simulink model "localPlanServer"  (R2024a)
settings: Solver=FixedStepDiscrete  StartTime=0.0  StopTime=inf  RelTol=1e-3
model workspace (MAT data in the model file):
  SL_ROS_VariableLengthArrays_MaxSizes.CommonInfo.ArrayTruncateAction = 'EmitWarning'
  SL_ROS_VariableLengthArrays_MaxSizes.MsgTypeMap = containers.Map
  SL_ROS_VariableLengthArrays_MaxSizes.MsgTypeMap.serialization.keys = {'std_msgs/Float64MultiArray', 'std_msgs/Int8MultiArray'}
  SL_ROS_VariableLengthArrays_MaxSizes.MsgTypeMap.serialization.values{1}.PropertyName = 'data'
  SL_ROS_VariableLengthArrays_MaxSizes.MsgTypeMap.serialization.values{1}.DataType = 'double'
  SL_ROS_VariableLengthArrays_MaxSizes.MsgTypeMap.serialization.values{1}.MaxLength = 30000
  SL_ROS_VariableLengthArrays_MaxSizes.MsgTypeMap.serialization.values{2}.PropertyName = 'data'
  SL_ROS_VariableLengthArrays_MaxSizes.MsgTypeMap.serialization.values{2}.DataType = 'int8'
  SL_ROS_VariableLengthArrays_MaxSizes.MsgTypeMap.serialization.values{2}.MaxLength = 1500000
  SL_ROS_VariableLengthArrays_MaxSizes.MsgTypeMap.serialization.uniformity = 0
  SL_ROS_VariableLengthArrays_MaxSizes.MsgTypeMap.serialization.keyType = 'char'
  SL_ROS_VariableLengthArrays_MaxSizes.MsgTypeMap.serialization.valueType = 'any'
undefined symbols (not defined in the file): nearestidx, needglobalreplan, needlocalreplan, optimizedpath, timestamps, velcmds
libraries: roshelperlib x6, simulink x2, ros2lib x2
settings Model: Creator=cstabile  LastModifiedBy=cstabile
settings OptimizationCC: EnhancedBackFolding=on  PassReuseOutputArgsAs=Individual arguments  ZeroExternalMemoryAtStartup=off  ZeroInternalMemoryAtStartup=off  MaxStackSize=64  OptimizeBlockOrder=speed  DifferentSizesBufferReuse=on  OptimizationCustomize=off  EfficientTunableParamExpr=on
settings DebuggingCC: ParameterTunabilityLossMsg=error
settings SFSimCC: MATLABDynamicMemAlloc=off
settings RTWCC: Description=Embedded Coder  SystemTargetFile=ert.tlc  HardwareBoard=Robot Operating System 2 (ROS 2)  TLCOptions="-aInlineSetEventsForThisBaseRateFcn=TLC_FALSE -aSuppressMultiTaskScheduler=TLC_FALSE  -aRateBasedStepFcn=0"  TemplateMakefile=ert_default_tmf  Toolchain=Colcon Tools  TargetLang=C++
settings CodeAppCC: ForceParamTrailComments=on  IgnoreCustomStorageClasses=off  OperatorAnnotations=on  SimulinkDataObjDesc=on  SFDataObjDesc=on  InsertBlockDesc=on
settings ERTTargetCC: CodeInterfacePackaging=C++ class  RootIOFormat=Structure reference

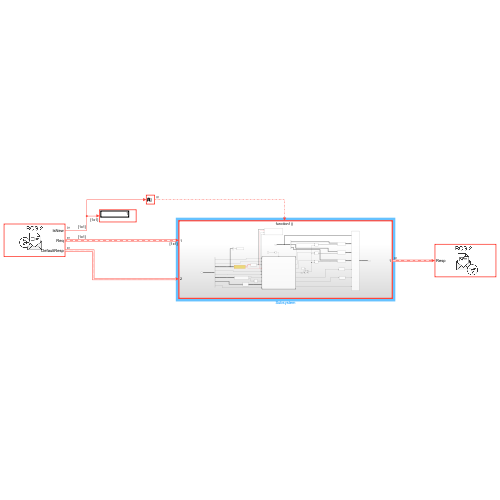
[thumbnail: Simulink's stored preview of the top-level diagram]
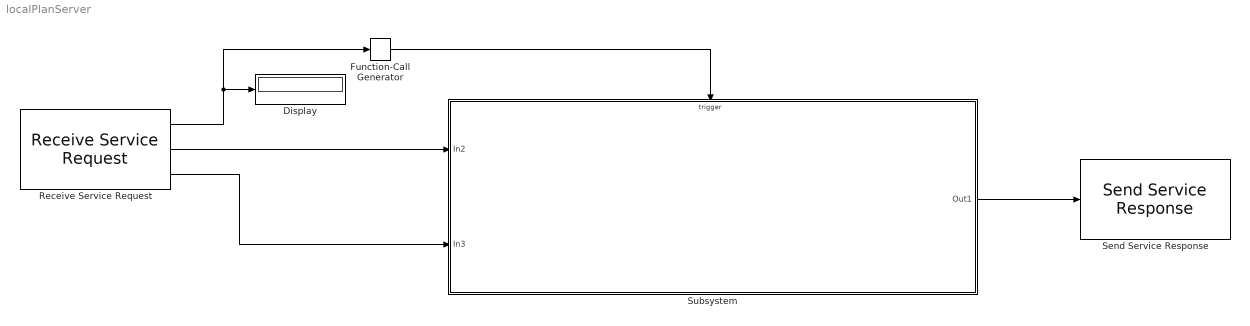
== system localPlanServer ==
  Display : Display
  Function-Call Generator : simulink/Ports & Subsystems/Function-Call Generator  sample_time=1  numberOfIterations=1  DisallowWideOutput=off  ShowEnablePort=on
  Receive Service Request : ros2lib/Receive Service Request  service=/planLocal  serviceType=offroad_msg/PlanLocal  SampleTime=-1  ShowDefaultRespOutput=on  BlockId=ServRec_localPlanServer_1  QOSHistory=Keep last  QOSDepth=1  QOSReliability=Reliable  QOSDurability=Volatile  QOSDeadline=Inf  QOSLifespan=Inf  QOSLiveliness=Automatic  QOSLeaseDuration=Inf  QOSAvoidROSNamespaceConventions=off
      settings: LibrarySourceBlock=ros2lib/Receive Request
  Send Service Response : ros2lib/Send Service Response  service=/planLocal  serviceType=offroad_msg/PlanLocal  BlockId=ServRec_localPlanServer_1
      settings: LibrarySourceBlock=ros2lib/Send Response
  Subsystem : Subsystem
  wires:
  Receive Service Request/1 -> Function-Call Generator/1, Display/1
  Function-Call Generator/1 -> Subsystem/Trigger
  Receive Service Request/2 -> Subsystem/1(In2)
  Receive Service Request/3 -> Subsystem/2(In3)
  Subsystem/1(Out1) -> Send Service Response/1

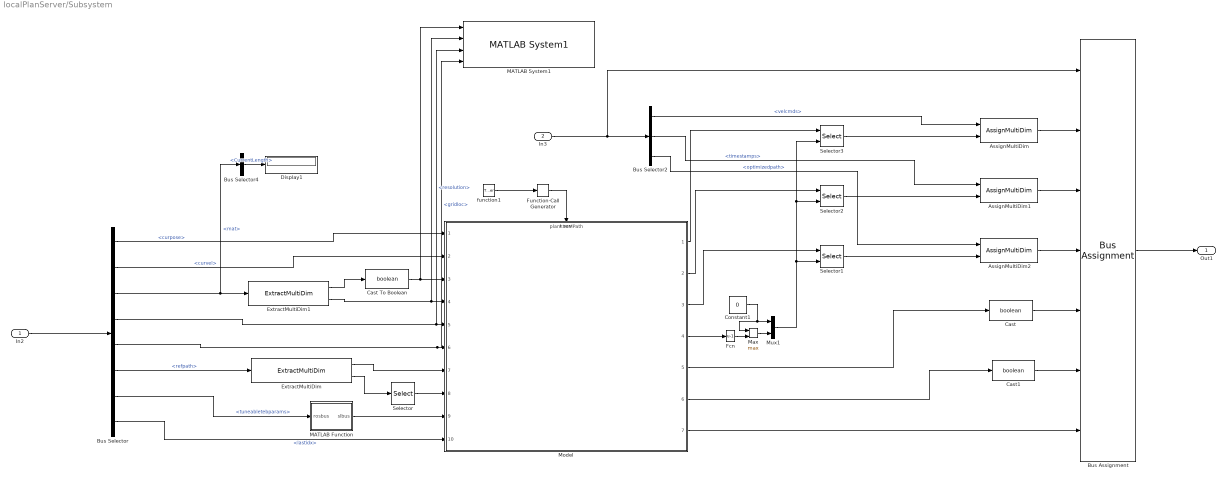
== system localPlanServer/Subsystem ==
  In2 : Inport
  In3 : Inport  Port=2
  function1 : TriggerPort  TriggerType=function-call  VariantControl=(inherit)  ShowOutputPort=on
  AssignMultiDim : roshelperlib/AssignMultiDim  SystemSampleTime=-1  VariantActivationTime=update diagram  AllowFlexibleInterface=on  Latency=0  AutoFrameSizeCalculation=off
  AssignMultiDim1 : roshelperlib/AssignMultiDim  SystemSampleTime=-1  VariantActivationTime=update diagram  AllowFlexibleInterface=on  Latency=0  AutoFrameSizeCalculation=off
  AssignMultiDim2 : roshelperlib/AssignMultiDim  SystemSampleTime=-1  VariantActivationTime=update diagram  AllowFlexibleInterface=on  Latency=0  AutoFrameSizeCalculation=off
  Bus Assignment : BusAssignment  AssignedSignals=velcmds,timestamps,optimizedpath,needlocalreplan,needglobalreplan,nearestidx
  Bus Selector : BusSelector  OutputSignals=curpose,curvel,mat,resolution,gridloc,refpath,tuneabletebparams,lastidx
  Bus Selector2 : BusSelector  OutputSignals=velcmds,timestamps,optimizedpath
  Bus Selector4 : BusSelector  OutputSignals=data_SL_Info.CurrentLength
  Cast : DataTypeConversion  OutDataTypeStr=boolean  SaturateOnIntegerOverflow=off  RndMeth=Floor
  Cast To Boolean : DataTypeConversion  OutDataTypeStr=boolean  SaturateOnIntegerOverflow=off  RndMeth=Floor
  Cast1 : DataTypeConversion  OutDataTypeStr=boolean  SaturateOnIntegerOverflow=off  RndMeth=Floor
  Constant1 : Constant  Value=0
  Display1 : Display
  ExtractMultiDim : roshelperlib/ExtractMultiDim  userDataType=double  dims=[10000 3]  isVarsize=on  varsizeDims=[1 0]  returnFixedTF=on
  ExtractMultiDim1 : roshelperlib/ExtractMultiDim  userDataType=int8  dims=[1201 1201]  isVarsize=on  varsizeDims=[1 1]  returnFixedTF=off
  Fcn : Fcn  Expr=u-1
  Function-Call Generator : simulink/Ports & Subsystems/Function-Call Generator  sample_time=1  numberOfIterations=1  DisallowWideOutput=off  ShowEnablePort=on
  MATLAB Function : MATLAB Function  TreatAsAtomicUnit=on
  MATLAB System1 : roshelperlib/MATLAB System1  MapType=SDF  IsEgo=off  DisplayVisual=on  SimulateUsing=Interpreted execution
  Max : MinMax  Function=max  Inputs=2
  Model : ModelReference  ModelNameDialog=planLocalPath.slx  SimulationMode=Normal  ModelReferenceVersion=1.7  TriggerPortName=function  TriggerPortTriggerType=function-call  TriggerPortStatesWhenEnabling=held
  Mux1 : Mux  Inputs=2
  Selector : Selector  InputPortWidth=2  IndexOptions=Index vector (dialog)  Indices=1  OutputSizes=1
  Selector1 : Selector  NumberOfDimensions=2  IndexMode=Zero-based  InputPortWidth=3  IndexOptions=Starting and ending indices (port),Select all  Indices=[1 3],1  OutputSizes=1,1
  Selector2 : Selector  NumberOfDimensions=2  IndexMode=Zero-based  InputPortWidth=3  IndexOptions=Starting and ending indices (port),Select all  Indices=[1 3],1  OutputSizes=1,1
  Selector3 : Selector  NumberOfDimensions=2  IndexMode=Zero-based  InputPortWidth=3  IndexOptions=Starting and ending indices (port),Select all  Indices=[1 3],1  OutputSizes=1,1
  Out1 : Outport
  wires:
  Bus Selector2/2 -> AssignMultiDim1/1  "<timestamps>"
  In3/1 -> Bus Assignment/1, Bus Selector2/1
  Model/4 -> Fcn/1
  Bus Selector/4 -> MATLAB System1/3, Model/5  "<resolution>"
  Bus Selector/5 -> MATLAB System1/4, Model/6  "<gridloc>"
  Bus Selector2/1 -> AssignMultiDim/1  "<velcmds>"
  In2/1 -> Bus Selector/1
  Max/1 -> Mux1/2
  ExtractMultiDim/2 -> Selector/1
  ExtractMultiDim1/2 -> MATLAB System1/2, Model/4
  Constant1/1 -> Max/1, Mux1/1
  Mux1/1 -> Selector1/2, Selector3/2, Selector2/2
  Bus Selector/6 -> ExtractMultiDim/1  "<refpath>"
  Selector1/1 -> AssignMultiDim2/2
  Bus Selector2/3 -> AssignMultiDim2/1  "<optimizedpath>"
  Bus Assignment/1 -> Out1/1
  Bus Selector/3 -> Bus Selector4/1, ExtractMultiDim1/1  "<mat>"
  AssignMultiDim1/1 -> Bus Assignment/3
  ExtractMultiDim/1 -> Model/7
  AssignMultiDim/1 -> Bus Assignment/2
  Selector/1 -> Model/8
  Selector2/1 -> AssignMultiDim1/2
  Model/6 -> Cast1/1
  Selector3/1 -> AssignMultiDim/2
  Model/2 -> Selector2/1
  Bus Selector/1 -> Model/1  "<curpose>"
  Model/5 -> Cast/1
  Cast To Boolean/1 -> MATLAB System1/1, Model/3
  Model/1 -> Selector3/1
  Cast1/1 -> Bus Assignment/6
  Cast/1 -> Bus Assignment/5
  ExtractMultiDim1/1 -> Cast To Boolean/1
  Fcn/1 -> Max/2
  AssignMultiDim2/1 -> Bus Assignment/4
  MATLAB Function/1(slbus) -> Model/9
  Model/3 -> Selector1/1
  Bus Selector4/1 -> Display1/1  "<CurrentLength>"
  function1/1 -> Function-Call Generator/1
  Function-Call Generator/1 -> Model/Trigger
  Model/7 -> Bus Assignment/7
  Bus Selector/2 -> Model/2  "<curvel>"
  Bus Selector/7 -> MATLAB Function/1(rosbus)  "<tuneabletebparams>"
  Bus Selector/8 -> Model/10  "<lastidx>"

== matlab function localPlanServer/Subsystem/MATLAB Function ==
  data: rosbus input; slbus output Bus: teb_bus
function slbus = fcn(rosbus)
    slbus.LookaheadTime = rosbus.lookaheadtime;
    slbus.ObstacleSafetyMargin = rosbus.obstaclesafetymargin;
    slbus.CostWeights_T.Time = rosbus.costweights.time;
    slbus.CostWeights_T.Smoothness = rosbus.costweights.smoothness;
    slbus.CostWeights_T.Obstacle = rosbus.costweights.obstacle;
    slbus.MinTurningRadius = rosbus.minturningradius;
    slbus.MaxVelocity = rosbus.maxvelocity(:)';
    slbus.MaxAcceleration = rosbus.maxacceleration(:)';
    slbus.MaxReverseVelocity = rosbus.maxreversevelocity;
end
